simulink model "said"  (R2024a)
settings: Solver=VariableStepAuto  StartTime=0.0  StopTime=inf  RelTol=1e-3
settings Model: Creator=pc  LastModifiedBy=pc

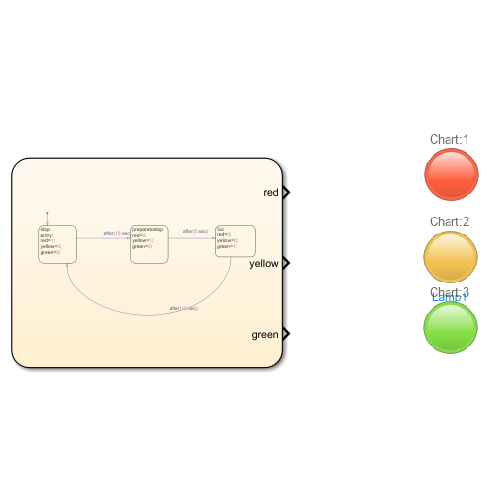
[thumbnail: Simulink's stored preview of the top-level diagram]
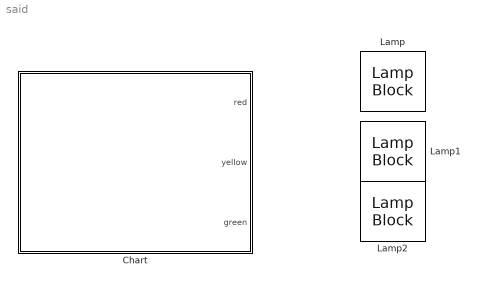
== system said ==
  Chart : Stateflow chart  TreatAsAtomicUnit=on
  Lamp : LampBlock
  Lamp1 : LampBlock
  Lamp2 : LampBlock

== stateflow chart said/Chart ==
  state stop
    entry:
    red=1;
    yellow=0;
    green=0;
  state preparetostop
    red=0;
    yellow=1;
    green=0;
  state Go
    red=0;
    yellow=0;
    green=1;
  (default) -> stop
  preparetostop -> Go : after(5,sec)
  stop -> preparetostop : after(15,sec)
  Go -> stop : after(15,sec)
  data: red output; yellow output; green output
